simulink model "sampleModel348"  (R2021b)
settings: Solver=VariableStepAuto  StartTime=0.0  StopTime=10.0  RelTol=1e-3
undefined symbols (not defined in the file or in its folder): DiscIntNeverNeededParam, Newton, Raphson
libraries: simulink x6
settings Model: Creator=user  LastModifiedBy=user

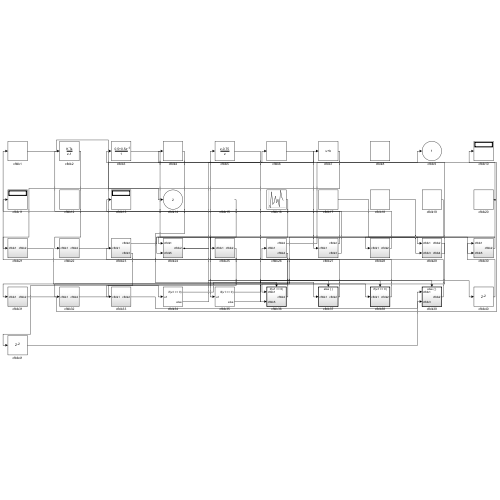
[thumbnail: Simulink's stored preview of the top-level diagram]
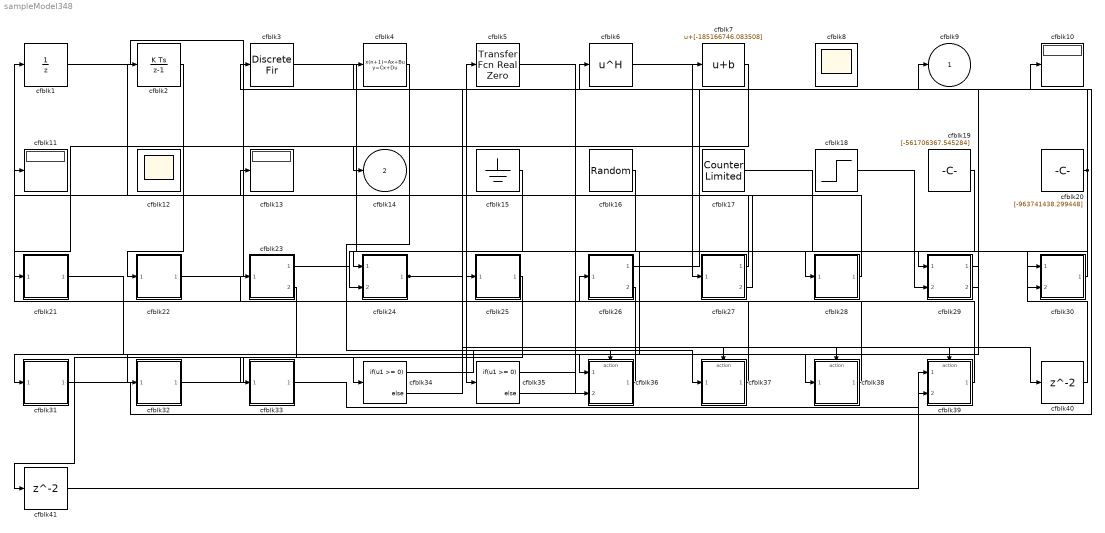
== system sampleModel348 ==
  cfblk1 : UnitDelay  HasFrameUpgradeWarning=on
  cfblk10 : Display
  cfblk11 : Display
  cfblk12 : Scope
      settings: Floating=on
  cfblk13 : Display
  cfblk15 : Ground
  cfblk16 : UniformRandomNumber  Minimum=[-3290051227.706295]  Maximum=[4258944118.806231]  Seed=[72617073.000000]  SampleTime=0.1
  cfblk17 : simulink/Sources/Counter Limited  uplimit=[154.000000]  tsamp=-1
  cfblk18 : Step  Time=[45.000000]  Before=[-895383784.704633]  After=[265334180.994879]  SampleTime=0
  cfblk19 : Constant  Value=[-561706367.545284]  SampleTime=1
  cfblk2 : DiscreteIntegrator  ICPrevOutput=DiscIntNeverNeededParam  ICPrevScaledInput=DiscIntNeverNeededParam
  cfblk20 : Constant  Value=[-963741438.299448]  SampleTime=1
  cfblk21 : Subsystem
  cfblk22 : Subsystem
  cfblk23 : Subsystem
  cfblk24 : Subsystem
  cfblk25 : Subsystem
  cfblk26 : Subsystem
  cfblk27 : Subsystem
  cfblk28 : Subsystem
  cfblk29 : Subsystem
  cfblk3 : DiscreteFir  SampleTime=1
  cfblk30 : Subsystem
  cfblk31 : Subsystem
  cfblk32 : Subsystem
  cfblk33 : Subsystem
  cfblk34 : If  IfExpression=u1 >= 0  SampleTime=1
  cfblk35 : If  IfExpression=u1 >= 0  SampleTime=1
  cfblk36 : Subsystem  TreatAsAtomicUnit=on
  cfblk37 : Subsystem  TreatAsAtomicUnit=on
  cfblk38 : Subsystem  TreatAsAtomicUnit=on
  cfblk39 : Subsystem  TreatAsAtomicUnit=on
  cfblk4 : DiscreteStateSpace
  cfblk40 : Delay  SampleTime=1
  cfblk41 : Delay  SampleTime=1
  cfblk5 : simulink/Discrete/Transfer Fcn Real Zero  ZeroZ=0.75  ICPrevInput=0.0  DoSatur=off
      settings: SourceProductBaseCode=SL
  cfblk6 : Math  Operator=hermitian  SaturateOnIntegerOverflow=on
  cfblk7 : Bias  Bias=[-185166746.083508]
  cfblk8 : Scope
      settings: Floating=on
  cfblk9 : Outport
  cfblk14 : Outport  Port=2
  wires:
  cfblk2/1 -> cfblk22/1(cfblk1)
  cfblk38/1(cfblk2) -> cfblk5/1
  cfblk26/1(cfblk2) -> cfblk9/1
  cfblk32/1(cfblk2) -> cfblk34/1
  cfblk33/1(cfblk2) -> cfblk39/1(cfblk1)
  cfblk30/1(cfblk2) -> cfblk24/1(cfblk1)
  cfblk4/1 -> cfblk37/1(cfblk1)
  cfblk6/1 -> cfblk27/1(cfblk1)
  cfblk36/1(cfblk2) -> cfblk26/1(cfblk1)
  cfblk3/1 -> cfblk35/1
  cfblk20/1 -> cfblk28/1(cfblk1), cfblk4/1
  cfblk16/1 -> cfblk25/1(cfblk1)
  cfblk19/1 -> cfblk36/1(cfblk1)
  cfblk25/1(cfblk2) -> cfblk33/1(cfblk1)
  cfblk17/1 -> cfblk29/1(cfblk1)
  cfblk24/1(cfblk2) -> cfblk6/1, cfblk40/1
  cfblk27/1(cfblk2) -> cfblk1/1
  cfblk1/1 -> cfblk14/1
  cfblk28/1(cfblk2) -> cfblk2/1
  cfblk22/1(cfblk2) -> cfblk7/1
  cfblk31/1(cfblk2) -> cfblk10/1
  cfblk15/1 -> cfblk24/2(cfblk5)
  cfblk29/1(cfblk2) -> cfblk32/1(cfblk1)
  cfblk37/1(cfblk2) -> cfblk11/1
  cfblk7/1 -> cfblk21/1(cfblk1)
  cfblk29/2(cfblk4) -> cfblk3/1
  cfblk5/1 -> cfblk36/2(cfblk5)
  cfblk23/1(cfblk2) -> cfblk30/2(cfblk5)
  cfblk26/2(cfblk4) -> cfblk31/1(cfblk1)
  cfblk21/1(cfblk2) -> cfblk38/1(cfblk1)
  cfblk27/2(cfblk3) -> cfblk13/1
  cfblk39/1(cfblk2) -> cfblk23/1(cfblk1)
  cfblk18/1 -> cfblk29/2(cfblk3)
  cfblk34/1 -> cfblk36/Action
  cfblk34/2 -> cfblk37/Action
  cfblk35/1 -> cfblk38/Action
  cfblk35/2 -> cfblk39/Action
  cfblk40/1 -> cfblk30/1(cfblk1)
  cfblk23/2(cfblk3) -> cfblk41/1
  cfblk41/1 -> cfblk39/2(cfblk3)

== system sampleModel348/cfblk21 ==
  cfblk1 : Inport
  cfblk3 : DiscreteFilter  SampleTime=1
  cfblk2 : Outport
  wires:
  cfblk1/1 -> cfblk3/1
  cfblk3/1 -> cfblk2/1

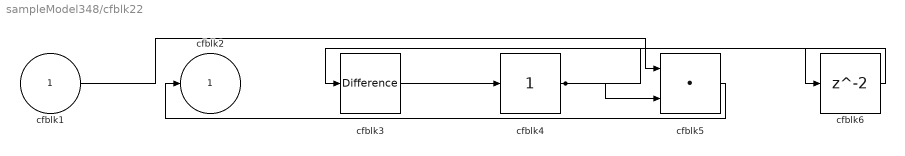
== system sampleModel348/cfblk22 ==
  cfblk1 : Inport
  cfblk3 : simulink/Discrete/Difference  ICPrevInput=0.0  OutMin=[]  OutMax=[]  OutDataTypeStr=Inherit: Inherit via back propagation  OutDataType=fixdt(1, 16)  OutScaling=2^-10  DoSatur=off
  cfblk4 : simulink/Math Operations/Slider Gain  gain=1  low=0  high=2
  cfblk5 : DotProduct  InputSameDT=on  OutDataTypeStr=Inherit: Inherit via internal rule
  cfblk6 : Delay  SampleTime=1
  cfblk2 : Outport
  wires:
  cfblk3/1 -> cfblk4/1
  cfblk4/1 -> cfblk5/2, cfblk6/1
  cfblk5/1 -> cfblk2/1
  cfblk1/1 -> cfblk5/1
  cfblk6/1 -> cfblk3/1

== system sampleModel348/cfblk23 ==
  cfblk1 : Inport
  cfblk2 : Outport
  cfblk3 : Outport  Port=2
  wires:
  cfblk1/1 -> cfblk3/1, cfblk2/1

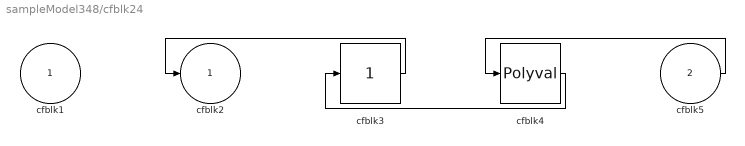
== system sampleModel348/cfblk24 ==
  cfblk1 : Inport
  cfblk5 : Inport  Port=2
  cfblk3 : simulink/Math Operations/Slider Gain  gain=1  low=0  high=2
  cfblk4 : Polyval  Coefs=[ +2.081618890e-019, -1.441693666e-014, +4.719686976e-010, -8.536869453e-006, +1.621573104e-001, -8.087801117e+001 ]
  cfblk2 : Outport
  wires:
  cfblk3/1 -> cfblk2/1
  cfblk4/1 -> cfblk3/1
  cfblk5/1 -> cfblk4/1

== system sampleModel348/cfblk25 ==
  cfblk1 : Inport
  cfblk3 : Rounding
  cfblk2 : Outport
  wires:
  cfblk1/1 -> cfblk3/1
  cfblk3/1 -> cfblk2/1

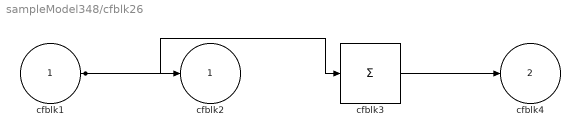
== system sampleModel348/cfblk26 ==
  cfblk1 : Inport
  cfblk3 : Sum  Inputs=+
  cfblk2 : Outport
  cfblk4 : Outport  Port=2
  wires:
  cfblk3/1 -> cfblk4/1
  cfblk1/1 -> cfblk2/1, cfblk3/1

== system sampleModel348/cfblk27 ==
  cfblk1 : Inport
  cfblk2 : Outport
  cfblk3 : Outport  Port=2
  wires:
  cfblk1/1 -> cfblk3/1, cfblk2/1

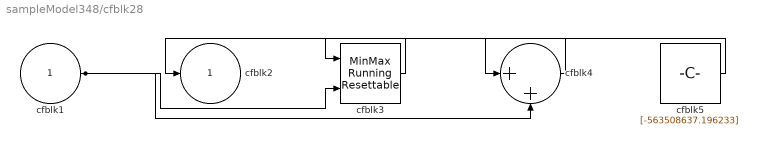
== system sampleModel348/cfblk28 ==
  cfblk1 : Inport
  cfblk3 : simulink/Math Operations/MinMax Running Resettable  Function=min  vinit=0.0
  cfblk4 : Sum  Inputs=|++
  cfblk5 : Constant  Value=[-563508637.196233]  SampleTime=1
  cfblk2 : Outport
  wires:
  cfblk5/1 -> cfblk4/1
  cfblk3/1 -> cfblk2/1
  cfblk1/1 -> cfblk4/2, cfblk3/2
  cfblk4/1 -> cfblk3/1

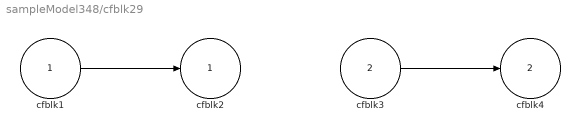
== system sampleModel348/cfblk29 ==
  cfblk1 : Inport
  cfblk3 : Inport  Port=2
  cfblk2 : Outport
  cfblk4 : Outport  Port=2
  wires:
  cfblk3/1 -> cfblk4/1
  cfblk1/1 -> cfblk2/1

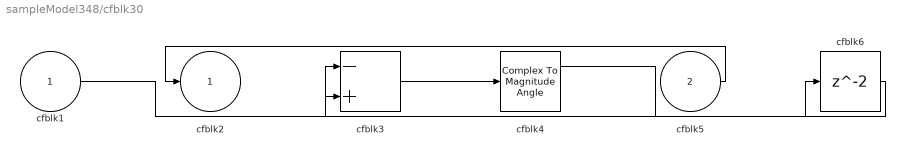
== system sampleModel348/cfblk30 ==
  cfblk1 : Inport
  cfblk5 : Inport  Port=2
  cfblk3 : Sum  Inputs=-+
  cfblk4 : ComplexToMagnitudeAngle
  cfblk6 : Delay  SampleTime=1
  cfblk2 : Outport
  wires:
  cfblk5/1 -> cfblk2/1
  cfblk1/1 -> cfblk3/1
  cfblk3/1 -> cfblk4/1
  cfblk4/1 -> cfblk6/1
  cfblk6/1 -> cfblk3/2

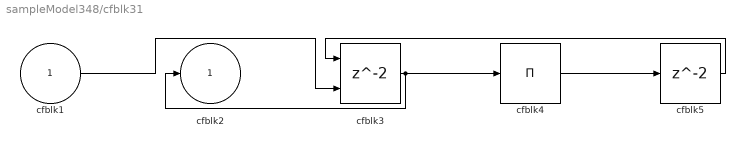
== system sampleModel348/cfblk31 ==
  cfblk1 : Inport
  cfblk3 : Delay  ShowEnablePort=on  SampleTime=1
      settings: InputPortMap=u0,e6
  cfblk4 : Product  Inputs=*
  cfblk5 : Delay  SampleTime=1
  cfblk2 : Outport
  wires:
  cfblk3/1 -> cfblk2/1, cfblk4/1
  cfblk1/1 -> cfblk3/2
  cfblk4/1 -> cfblk5/1
  cfblk5/1 -> cfblk3/1

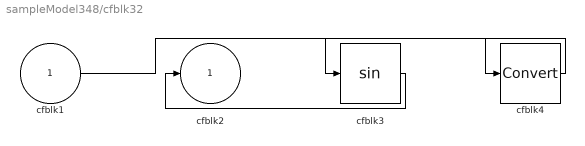
== system sampleModel348/cfblk32 ==
  cfblk1 : Inport
  cfblk3 : Trigonometry
  cfblk4 : DataTypeConversion
  cfblk2 : Outport
  wires:
  cfblk3/1 -> cfblk2/1
  cfblk1/1 -> cfblk4/1
  cfblk4/1 -> cfblk3/1

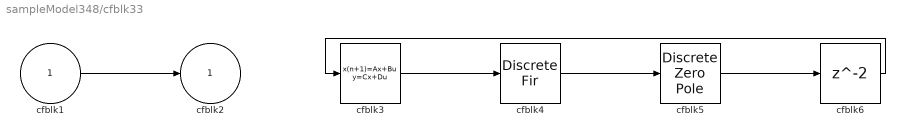
== system sampleModel348/cfblk33 ==
  cfblk1 : Inport
  cfblk3 : DiscreteStateSpace
  cfblk4 : DiscreteFir  SampleTime=1
  cfblk5 : DiscreteZeroPole  Poles=[0 0.5]  Gain=1
  cfblk6 : Delay  SampleTime=1
  cfblk2 : Outport
  wires:
  cfblk3/1 -> cfblk4/1
  cfblk4/1 -> cfblk5/1
  cfblk1/1 -> cfblk2/1
  cfblk5/1 -> cfblk6/1
  cfblk6/1 -> cfblk3/1

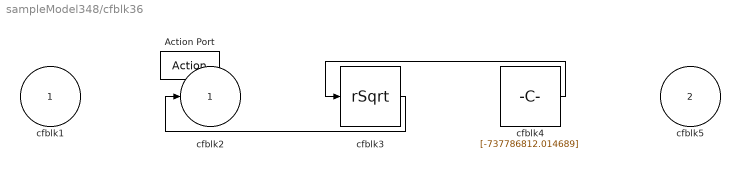
== system sampleModel348/cfblk36 ==
  cfblk1 : Inport
  cfblk5 : Inport  Port=2
  Action Port : ActionPort  ActionPortLabel=if(u1 >= 0)
  cfblk3 : Sqrt  Operator=rSqrt  AlgorithmType=Newton-Raphson  SaturateOnIntegerOverflow=on
  cfblk4 : Constant  Value=[-737786812.014689]  SampleTime=1
  cfblk2 : Outport
  wires:
  cfblk3/1 -> cfblk2/1
  cfblk4/1 -> cfblk3/1

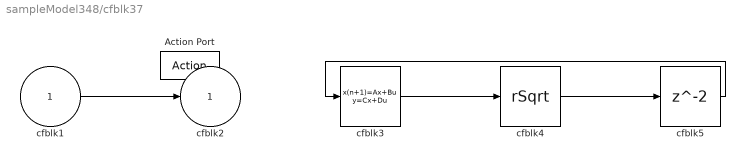
== system sampleModel348/cfblk37 ==
  cfblk1 : Inport
  Action Port : ActionPort  ActionPortLabel=else
  cfblk3 : DiscreteStateSpace  SampleTime=-1
  cfblk4 : Sqrt  Operator=rSqrt  AlgorithmType=Newton-Raphson  SaturateOnIntegerOverflow=on
  cfblk5 : Delay
  cfblk2 : Outport
  wires:
  cfblk3/1 -> cfblk4/1
  cfblk1/1 -> cfblk2/1
  cfblk4/1 -> cfblk5/1
  cfblk5/1 -> cfblk3/1

== system sampleModel348/cfblk38 ==
  cfblk1 : Inport
  Action Port : ActionPort  ActionPortLabel=if(u1 >= 0)
  cfblk3 : Rounding
  cfblk2 : Outport
  wires:
  cfblk1/1 -> cfblk2/1, cfblk3/1

== system sampleModel348/cfblk39 ==
  cfblk1 : Inport
  cfblk3 : Inport  Port=2
  Action Port : ActionPort  ActionPortLabel=else
  cfblk2 : Outport
  wires:
  cfblk1/1 -> cfblk2/1
